simulink model "oven"  (R2016a)
settings: Solver=VariableStepAuto  StartTime=0.0  StopTime=10.0  RelTol=1e-3
values from neighbouring files (symbols this model uses):
  a1 = T1+T2    (= 150)    [step_response_analysis.m]
  a2 = T1*T2    (= 3600)    [step_response_analysis.m]
  Kd = 0    [step_response_analysis.m]
  Ki = Kp / Tn    (= 0.000133484478836)    [step_response_analysis.m]
  Kp = 0.65 * (Tg / (Tu*Ks))    (= 0.0248281130634)    [step_response_analysis.m]
  Ks = 340    [step_response_analysis.m]
libraries: simulink x2
settings Model: Creator=Julian  LastModifiedBy=Julian
settings DataIOCC: SaveFormat=Array
settings GRTTargetCC: GeneratePreprocessorConditionals=Use local settings

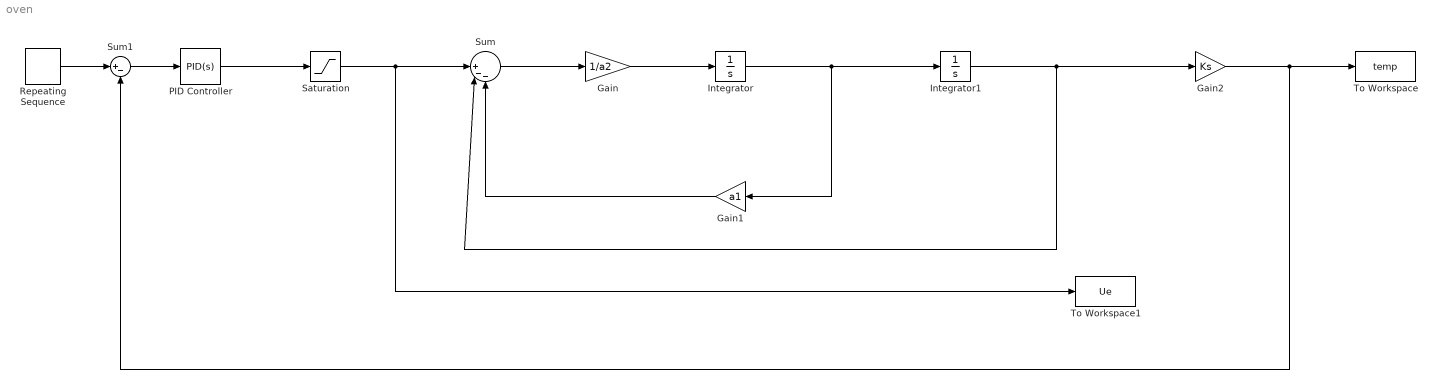
== system oven ==
  Gain : Gain  Gain=1/a2
  Gain1 : Gain  Gain=a1
  Gain2 : Gain  Gain=Ks
  Integrator : Integrator
  Integrator1 : Integrator
  PID Controller : simulink/Continuous/PID Controller  Controller=PID  TimeDomain=Continuous-time  SampleTime=-1  IntegratorMethod=Forward Euler  FilterMethod=Forward Euler  Form=Parallel  UseFilter=on  ControllerParametersSource=internal  P=Kp  I=Ki  D=Kd  N=100  InitialConditionSource=internal  InitialConditionForIntegrator=0  InitialConditionForFilter=0  ExternalReset=none  LimitOutput=off  UpperSaturationLimit=inf  LowerSaturationLimit=-inf  LinearizeAsGain=on  AntiWindupMode=none  Kb=1  TrackingMode=off  Kt=1  PParamMin=[]  PParamMax=[]  IParamMin=[]  IParamMax=[]  DParamMin=[]  DParamMax=[]  NParamMin=[]  NParamMax=[]  KbParamMin=[]  KbParamMax=[]  KtParamMin=[]  KtParamMax=[]  POutMin=[]  POutMax=[]  IOutMin=[]  IOutMax=[]  DOutMin=[]  DOutMax=[]  NOutMin=[]  NOutMax=[]  KbOutMin=[]  KbOutMax=[]  KtOutMin=[]  KtOutMax=[]  IntegratorOutMin=[]  IntegratorOutMax=[]  FilterOutMin=[]  FilterOutMax=[]  SumOutMin=[]  SumOutMax=[]  SumI1OutMin=[]  SumI1OutMax=[]  SumI2OutMin=[]  SumI2OutMax=[]  SumI3OutMin=[]  SumI3OutMax=[]  SumDOutMin=[]  SumDOutMax=[]  SaturationOutMin=[]  SaturationOutMax=[]  IntegratorContinuousStateAttributes=''  IntegratorStateMustResolveToSignalObject=off  IntegratorRTWStateStorageClass=Auto  FilterContinuousStateAttributes=''  FilterStateMustResolveToSignalObject=off  FilterRTWStateStorageClass=Auto  DifferentiatorICPrevScaledInput=0  DifferentiatorOutMin=[]  DifferentiatorOutMax=[]
  Repeating Sequence : simulink/Sources/Repeating Sequence  rep_seq_t=reflow_times  rep_seq_y=reflow_temps
  Saturation : Saturate  UpperLimit=1  LowerLimit=0
  Sum : Sum  Inputs=||+--
  Sum1 : Sum  Inputs=|+-
  To Workspace : ToWorkspace  VariableName=temp  SampleTime=-1
  To Workspace1 : ToWorkspace  VariableName=Ue  SampleTime=-1
  wires:
  Sum/1 -> Gain/1
  Gain/1 -> Integrator/1
  Integrator/1 -> Gain1/1, Integrator1/1
  Gain1/1 -> Sum/3
  Integrator1/1 -> Gain2/1, Sum/2
  Gain2/1 -> Sum1/2, To Workspace/1
  Sum1/1 -> PID Controller/1
  Repeating Sequence/1 -> Sum1/1
  PID Controller/1 -> Saturation/1
  Saturation/1 -> To Workspace1/1, Sum/1
